simulink model "wtLinModelSimulink"  (R2021b)
settings: Solver=VariableStepAuto  StartTime=0.0  StopTime=10.0  RelTol=1e-3
undefined symbols (not defined in the file): A, B, C, u_op, x_init, x_op
settings Model: Creator=martin  LastModifiedBy=martin

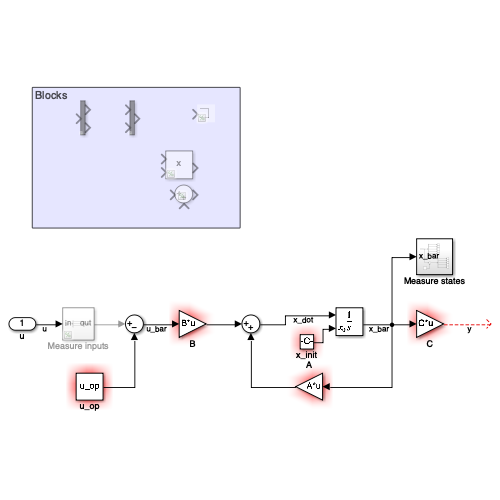
[thumbnail: Simulink's stored preview of the top-level diagram]
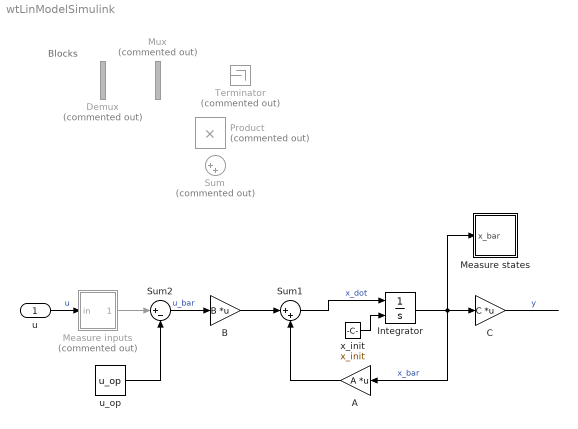
== system wtLinModelSimulink ==
  note: Blocks
  u : Inport
  A : Gain  Gain=A  Multiplication=Matrix(K*u)
  B : Gain  Gain=B  Multiplication=Matrix(K*u)
  C : Gain  Gain=C  Multiplication=Matrix(K*u)
  Demux : Demux  Commented=on  Outputs=2
  Integrator : Integrator  InitialConditionSource=external
  Measure inputs : Subsystem  Commented=on
  Measure states : Subsystem
  Mux : Mux  Commented=on  Inputs=2
  Product : Product  Commented=on
  Sum : Sum  Commented=on  Inputs=|++
  Sum1 : Sum  Inputs=|++
  Sum2 : Sum  Inputs=|+-
  Terminator : Terminator  Commented=on
  u_op : Constant  Value=u_op
  x_init : Constant  Value=x_init
  wires:
  A/1 -> Sum1/2
  Sum1/1 -> Integrator/1  "x_dot"
  B/1 -> Sum1/1
  u/1 -> Measure inputs/1(in)  "u"
  x_init/1 -> Integrator/2
  Integrator/1 -> Measure states/1(x_bar), C/1, A/1  "x_bar"
  Measure inputs/1(out) -> Sum2/1
  C/1 -> ?  "y"
  Sum2/1 -> B/1  "u_bar"
  u_op/1 -> Sum2/2

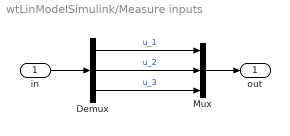
== system wtLinModelSimulink/Measure inputs ==
  in : Inport
  Demux : Demux  Outputs=3
  Mux : Mux  Inputs=3
  out : Outport
  wires:
  Demux/1 -> Mux/1  "u_1"
  Demux/2 -> Mux/2  "u_2"
  Demux/3 -> Mux/3  "u_3"
  Mux/1 -> out/1
  in/1 -> Demux/1

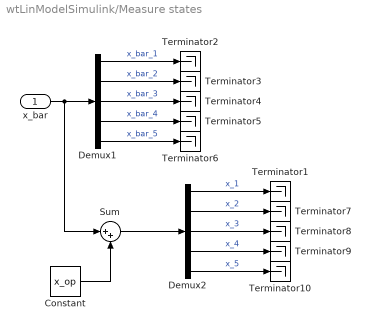
== system wtLinModelSimulink/Measure states ==
  x_bar : Inport
  Constant : Constant  Value=x_op
  Demux1 : Demux  Outputs=5
  Demux2 : Demux  Outputs=5
  Sum : Sum  Inputs=|++
  Terminator{1..10} (10 alike) : Terminator
  wires:
  Demux1/5 -> Terminator6/1  "x_bar_5"
  Demux1/3 -> Terminator4/1  "x_bar_3"
  Demux1/1 -> Terminator2/1  "x_bar_1"
  Demux1/2 -> Terminator3/1  "x_bar_2"
  Demux1/4 -> Terminator5/1  "x_bar_4"
  x_bar/1 -> Sum/1, Demux1/1
  Demux2/3 -> Terminator8/1  "x_3"
  Demux2/2 -> Terminator7/1  "x_2"
  Demux2/1 -> Terminator1/1  "x_1"
  Demux2/4 -> Terminator9/1  "x_4"
  Demux2/5 -> Terminator10/1  "x_5"
  Sum/1 -> Demux2/1
  Constant/1 -> Sum/2
